simulink model "soar_interface_unit_test"  (R2018b)
settings: Solver=ode4  StartTime=0.0  StopTime=60  FixedStep=simParams.sample_time_s  RelTol=1e-3
values from neighbouring files (symbols this model uses):
  hw_in = [2.1259e-6;5.8341e-6;-8.6055e-7]    [soar_interface_unit_test_init.m]
  MET_epoch = simParams.time.epoch_utc_s    [soar_interface_unit_test_init.m]
  omega_cmd = [ 0.0; 0.0; 0.0 ]    [soar_interface_unit_test_init.m]
  omega_in = [0.00012082;0.00014607;0.021011]    [soar_interface_unit_test_init.m]
  quat_cmd = [ 1.0; 0.0; 0.0; 0.0 ]    [soar_interface_unit_test_init.m]
  quat_in = [ cosd(ang/2); sind(ang/2).*ax ]    [soar_interface_unit_test_init.m]
  sc_mode = 8    [soar_interface_unit_test_init.m]
  sI_unit = [ 1.0; 0.0; 0.0 ]    [soar_interface_unit_test_init.m]
undefined symbols (not defined in the file or in its folder): fswParams, quat_kinematics_lib, rigid_body_dynamics_lib, simParams
libraries: simulink x2, quat_err_lib x1, quat_degerr_check x1, quat_degerr_lib x1, sharedutil x1, quat_rectify_lib x1, vrlib x1, aerolibutil x1, soar_interface_lib x1
settings Model: Creator=taylorreynolds  LastModifiedBy=Taylor
settings DebuggingCC: SingleTaskRateTransMsg=error
settings SFSimCC: SimUseLocalCustomCode=off
settings RTWCC: GenerateReport=on  RTWUseLocalCustomCode=off  LaunchReport=on
settings CodeAppCC: StateflowObjectComments=on

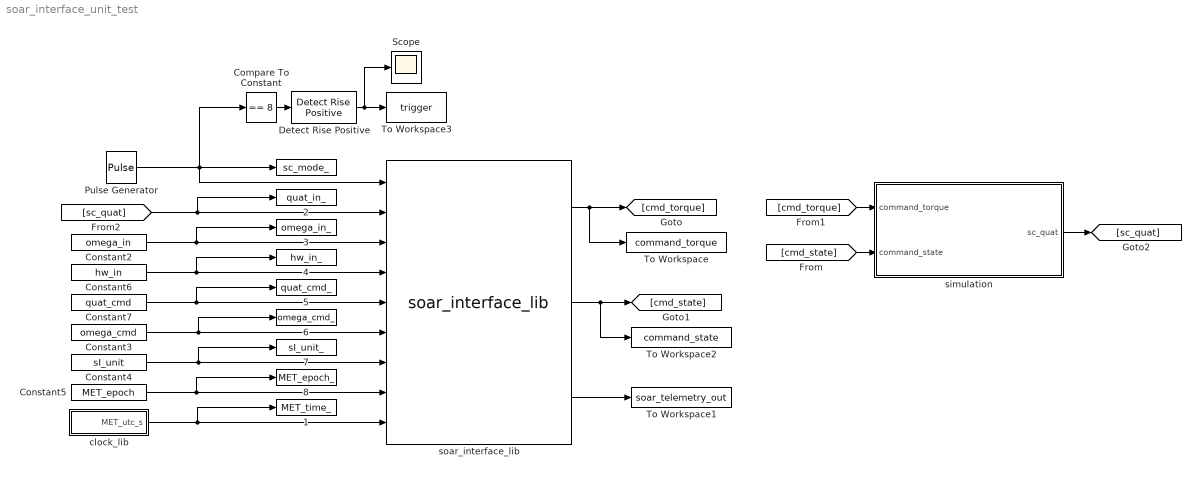
== system soar_interface_unit_test ==
  " " : ToWorkspace  VariableName=sc_mode_  SaveFormat=Timeseries  SampleTime=-1
  " 1" : ToWorkspace  VariableName=MET_time_  SaveFormat=Timeseries  SampleTime=-1
  " 2" : ToWorkspace  VariableName=quat_in_  SaveFormat=Timeseries  SampleTime=-1
  " 3" : ToWorkspace  VariableName=omega_in_  SaveFormat=Timeseries  SampleTime=-1
  " 4" : ToWorkspace  VariableName=hw_in_  SaveFormat=Timeseries  SampleTime=-1
  " 5" : ToWorkspace  VariableName=quat_cmd_  SaveFormat=Timeseries  SampleTime=-1
  " 6" : ToWorkspace  VariableName=omega_cmd_  SaveFormat=Timeseries  SampleTime=-1
  " 7" : ToWorkspace  VariableName=sI_unit_  SaveFormat=Timeseries  SampleTime=-1
  " 8" : ToWorkspace  VariableName=MET_epoch_  SaveFormat=Timeseries  SampleTime=-1
  Compare To Constant : simulink/Logic and Bit Operations/Compare To Constant  relop===  const=8  OutDataTypeStr=boolean
  Constant2 : Constant  Value=omega_in  SampleTime=-1
  Constant3 : Constant  Value=omega_cmd  SampleTime=-1
  Constant4 : Constant  Value=sI_unit  SampleTime=-1
  Constant5 : Constant  Value=MET_epoch  SampleTime=-1
  Constant6 : Constant  Value=hw_in  SampleTime=-1
  Constant7 : Constant  Value=quat_cmd  SampleTime=-1
  Detect Rise Positive : simulink/Logic and Bit Operations/Detect Rise Positive  vinit=0  OutDataTypeStr=boolean
  Pulse Generator : DiscretePulseGenerator  PulseType=Time based  Amplitude=sc_mode  Period=120  PulseWidth=5  SampleTime=simParams.sample_time_s
  Scope : Scope
  To Workspace : ToWorkspace  VariableName=command_torque  SampleTime=-1
  To Workspace1 : ToWorkspace  VariableName=soar_telemetry_out  SaveFormat=Timeseries  SampleTime=-1
  To Workspace2 : ToWorkspace  VariableName=command_state  SampleTime=-1
  To Workspace3 : ToWorkspace  VariableName=trigger  SampleTime=-1
  clock_lib : Subsystem
  simulation : Subsystem
  soar_interface_lib : soar_interface_lib/soar_interface_lib  SystemSampleTime=-1
  wires:
  Constant5/1 -> soar_interface_lib/8, " 8"/1
  soar_interface_lib/1 -> [cmd_torque], To Workspace/1
  soar_interface_lib/3 -> To Workspace1/1
  Constant6/1 -> soar_interface_lib/4, " 4"/1
  Constant7/1 -> soar_interface_lib/5, " 5"/1
  Constant4/1 -> soar_interface_lib/7, " 7"/1
  Constant2/1 -> soar_interface_lib/3, " 3"/1
  [sc_quat] -> soar_interface_lib/2, " 2"/1
  soar_interface_lib/2 -> To Workspace2/1, [cmd_state]
  [cmd_torque] -> simulation/1(command_torque)
  [cmd_state] -> simulation/2("command_state ")
  Constant3/1 -> soar_interface_lib/6, " 6"/1
  simulation/1(sc_quat) -> [sc_quat]
  Pulse Generator/1 -> soar_interface_lib/1, Compare To Constant/1, " "/1
  Compare To Constant/1 -> Detect Rise Positive/1
  Detect Rise Positive/1 -> Scope/1, To Workspace3/1
  clock_lib/1(MET_utc_s) -> soar_interface_lib/9, " 1"/1

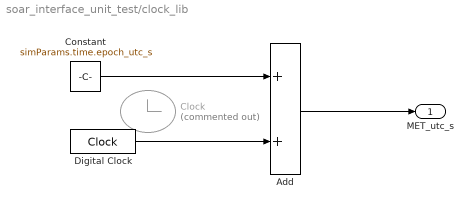
== system soar_interface_unit_test/clock_lib ==
  Add : Sum
  Clock : Clock  Commented=on
  Constant : Constant  Value=simParams.time.epoch_utc_s
  Digital Clock : DigitalClock  SampleTime=simParams.sample_time_s
  MET_utc_s : Outport
  wires:
  Digital Clock/1 -> Add/2
  Constant/1 -> Add/1
  Add/1 -> MET_utc_s/1

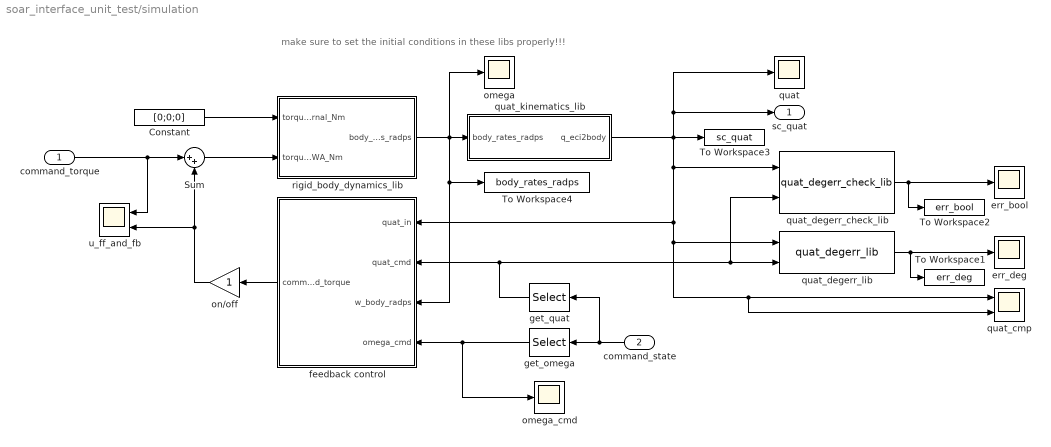
== system soar_interface_unit_test/simulation ==
  note: make sure to set the initial conditions in these libs properly!!!
  command_torque : Inport
  "command_state " : Inport  Port=2
  Constant : Constant  Value=[0;0;0]
  Sum : Sum  Inputs=|++
  To Workspace1 : ToWorkspace  VariableName=err_deg  SampleTime=-1
  To Workspace2 : ToWorkspace  VariableName=err_bool  SampleTime=-1
  To Workspace3 : ToWorkspace  VariableName=sc_quat  SampleTime=-1
  To Workspace4 : ToWorkspace  VariableName=body_rates_radps  SampleTime=-1
  err_bool : Scope
  err_deg : Scope
  feedback control : Subsystem
  get_omega : Selector  InputPortWidth=10  IndexOptions=Index vector (dialog)  Indices=[5 6 7]  OutputSizes=1
  get_quat : Selector  InputPortWidth=10  IndexOptions=Index vector (dialog)  Indices=[1 2 3 4]  OutputSizes=1
  omega : Scope
  omega_cmd : Scope
  on/off : Gain
  quat : Scope
  quat_cmp : Scope  NumInputPorts=2
  quat_degerr_check_lib : quat_degerr_check/quat_degerr_check_lib  point_tol=1
  quat_degerr_lib : quat_degerr_lib/quat_degerr_lib  SystemSampleTime=-1
  quat_kinematics_lib : Subsystem  AncestorBlock=quat_kinematics_lib/quat_kinematics_lib
  rigid_body_dynamics_lib : Subsystem  AncestorBlock=rigid_body_dynamics_lib/rigid_body_dynamics_lib
  u_ff_and_fb : Scope  NumInputPorts=2
  sc_quat : Outport
  wires:
  rigid_body_dynamics_lib/1(body_rates_radps) -> quat_kinematics_lib/1(body_rates_radps), feedback control/3(w_body_radps), To Workspace4/1, omega/1
  Constant/1 -> rigid_body_dynamics_lib/1(torque_external_Nm)
  get_quat/1 -> quat_degerr_check_lib/2, quat_degerr_lib/2, feedback control/2(quat_cmd)
  quat_degerr_check_lib/1 -> To Workspace2/1, err_bool/1
  quat_kinematics_lib/1(q_eci2body) -> sc_quat/1, quat/1, quat_cmp/2, quat_cmp/1, quat_degerr_lib/1, feedback control/1(quat_in), quat_degerr_check_lib/1, To Workspace3/1
  "command_state "/1 -> get_quat/1, get_omega/1
  Sum/1 -> rigid_body_dynamics_lib/2(torque_RWA_Nm)
  get_omega/1 -> omega_cmd/1, feedback control/4(omega_cmd)
  command_torque/1 -> u_ff_and_fb/1, Sum/1
  feedback control/1(command_torque) -> on/off/1
  on/off/1 -> u_ff_and_fb/2, Sum/2
  quat_degerr_lib/1 -> To Workspace1/1, err_deg/1

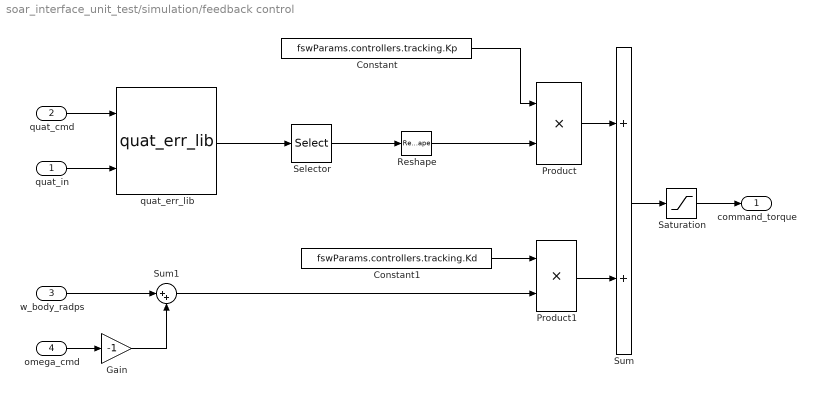
== system soar_interface_unit_test/simulation/feedback control ==
  quat_in : Inport
  quat_cmd : Inport  Port=2
  w_body_radps : Inport  Port=3
  omega_cmd : Inport  Port=4
  Constant : Constant  Value=fswParams.controllers.tracking.Kp
  Constant1 : Constant  Value=fswParams.controllers.tracking.Kd
  Gain : Gain  Gain=-1
  Product : Product
  Product1 : Product
  Reshape : Reshape
  Saturation : Saturate  UpperLimit=simParams.actuators.rwa.max_torque_Nm  LowerLimit=-simParams.actuators.rwa.max_torque_Nm
  Selector : Selector  InputPortWidth=4  IndexOptions=Index vector (dialog)  Indices=[2 3 4]  OutputSizes=1
  Sum : Sum
  Sum1 : Sum  Inputs=|++
  quat_err_lib : quat_err_lib/quat_err_lib  SystemSampleTime=-1
  command_torque : Outport
  wires:
  Selector/1 -> Reshape/1
  Sum1/1 -> Product1/2
  Gain/1 -> Sum1/2
  omega_cmd/1 -> Gain/1
  w_body_radps/1 -> Sum1/1
  Saturation/1 -> command_torque/1
  Product1/1 -> Sum/2
  Product/1 -> Sum/1
  Constant/1 -> Product/1
  Constant1/1 -> Product1/1
  Sum/1 -> Saturation/1
  quat_cmd/1 -> quat_err_lib/1
  quat_in/1 -> quat_err_lib/2
  quat_err_lib/1 -> Selector/1
  Reshape/1 -> Product/2

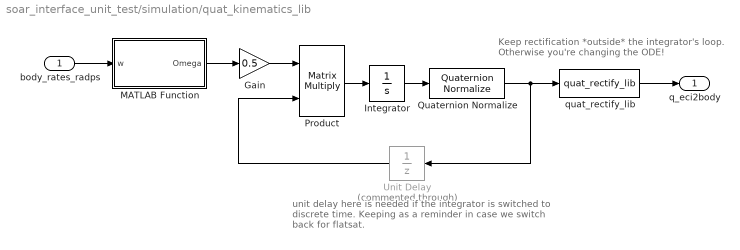
== system soar_interface_unit_test/simulation/quat_kinematics_lib ==
  note: unit delay here is needed if the integrator is
      | switched to discrete time. Keeping as a reminder
      | in case we switch back for flatsat.
  note: Keep rectification *outside* the integrator's
      | loop. Otherwise you're changing the ODE!
  body_rates_radps : Inport
  Gain : Gain  Gain=0.5
  Integrator : Integrator  InitialCondition=quat_in
  MATLAB Function : MATLAB Function  TreatAsAtomicUnit=on
  Product : Product  Multiplication=Matrix(*)
  Quaternion Normalize : sharedutil/Quaternion Normalize  aMode=aMode
      settings: SourceProductName=Aerospace Blockset  SourceProductBaseCode=AE
  Unit Delay : UnitDelay  Commented=through  InitialCondition=simParams.initialConditions.q_eci2body  SampleTime=-1
  quat_rectify_lib : quat_rectify_lib/quat_rectify_lib
  q_eci2body : Outport
  wires:
  quat_rectify_lib/1 -> q_eci2body/1
  Quaternion Normalize/1 -> quat_rectify_lib/1, Unit Delay/1
  Unit Delay/1 -> Product/2
  Gain/1 -> Product/1
  Product/1 -> Integrator/1
  MATLAB Function/1(Omega) -> Gain/1
  body_rates_radps/1 -> MATLAB Function/1(w)
  Integrator/1 -> Quaternion Normalize/1

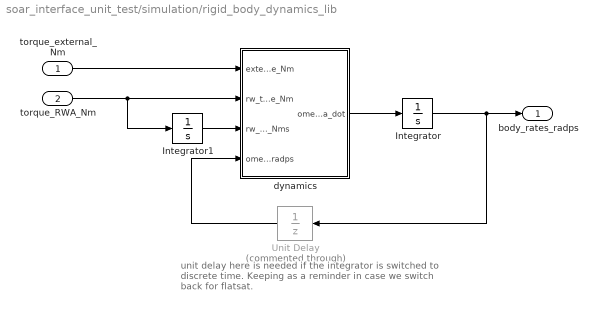
== system soar_interface_unit_test/simulation/rigid_body_dynamics_lib ==
  note: unit delay here is needed if the integrator is
      | switched to discrete time. Keeping as a reminder
      | in case we switch back for flatsat.
  torque_external_Nm : Inport
  torque_RWA_Nm : Inport  Port=2
  Integrator : Integrator  InitialCondition=omega_in
  Integrator1 : Integrator  InitialCondition=hw_in
  Unit Delay : UnitDelay  Commented=through  InitialCondition=simParams.initialConditions.w_body_radps  SampleTime=-1
  dynamics : Subsystem
  body_rates_radps : Outport
  wires:
  Unit Delay/1 -> dynamics/4(omega_radps)
  dynamics/1(omega_dot) -> Integrator/1
  Integrator1/1 -> dynamics/3(rw_momentum_Nms)
  torque_external_Nm/1 -> dynamics/1(external_torque_Nm)
  Integrator/1 -> body_rates_radps/1, Unit Delay/1
  torque_RWA_Nm/1 -> dynamics/2(rw_torque_Nm), Integrator1/1

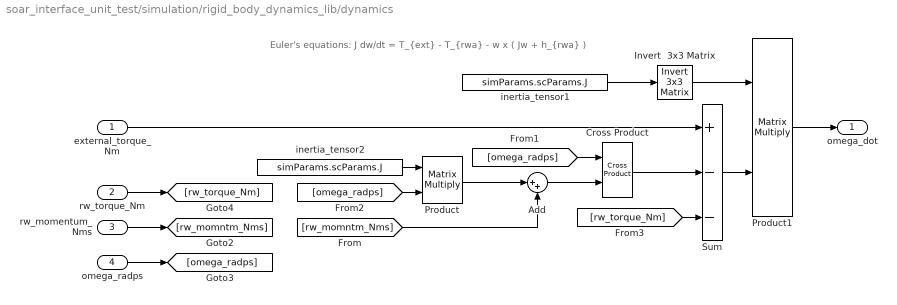
== system soar_interface_unit_test/simulation/rigid_body_dynamics_lib/dynamics ==
  note: Euler's equations: J dw/dt = T_{ext} - T_{rwa} - w x ( Jw + h_{rwa} )
  external_torque_Nm : Inport
  rw_torque_Nm : Inport  Port=2
  rw_momentum_Nms : Inport  Port=3
  omega_radps : Inport  Port=4
  Add : Sum  Inputs=|++
  Cross Product : vrlib/Utilities/Cross Product
      settings: SourceProductBaseCode=VR
  Invert  3x3 Matrix : aerolibutil/Invert  3x3 Matrix
  Product : Product  Multiplication=Matrix(*)  RndMeth=Zero
  Product1 : Product  Multiplication=Matrix(*)  RndMeth=Zero
  Sum : Sum  Inputs=+--
  inertia_tensor1 : Constant  Value=simParams.scParams.J  SampleTime=simParams.sample_time_s
  inertia_tensor2 : Constant  Value=simParams.scParams.J  SampleTime=simParams.sample_time_s
  omega_dot : Outport
  wires:
  [rw_torque_Nm] -> Sum/3
  [omega_radps] -> Product/2
  [omega_radps] -> Cross Product/1
  [rw_momntm_Nms] -> Add/2
  rw_momentum_Nms/1 -> [rw_momntm_Nms]
  external_torque_Nm/1 -> Sum/1
  omega_radps/1 -> [omega_radps]
  inertia_tensor2/1 -> Product/1
  Sum/1 -> Product1/2
  Product1/1 -> omega_dot/1
  Invert  3x3 Matrix/1 -> Product1/1
  inertia_tensor1/1 -> Invert  3x3 Matrix/1
  Cross Product/1 -> Sum/2
  Product/1 -> Add/1
  Add/1 -> Cross Product/2
  rw_torque_Nm/1 -> [rw_torque_Nm]

== matlab function soar_interface_unit_test/simulation/quat_kinematics_lib/MATLAB Function ==
  data: w input; Omega output
function Omega = q_skew_star(w)
%#codegen
Omega = [ 0.0,  -w(1), -w(2), -w(3);
          w(1),  0.0,   w(3), -w(2);
          w(2), -w(3),  0.0,   w(1);
          w(3),  w(2), -w(1),  0.0 ];
end
